simulink model "rx2"  (R2022b)
settings: Solver=FixedStepDiscrete  StartTime=0.0  StopTime=3.3E6  FixedStep=1  RelTol=1e-3  EnableMultiTasking=on
model workspace (MAT data in the model file):
  mwTaskManagerKernelLatency = 0
undefined symbols (not defined in the file or in its folder): Add, jsin, magnitude, rom_pilot_conj_tt, Shift
libraries: hdlsllib x3231, whdlutilities x525, simulink x260, whdlmod x112, whdledac x26, dsphdlmathfun2 x24, commchan3 x1
(part 39 of 59)

== system rx2/demode1/chan_est1/Subsystem/HDL_DUT1/H_est ==
  H_result_in : Inport
      settings: SignalType=complex
  H_ctrl_in : Inport  Port=2  OutDataTypeStr=Bus: samplecontrol
  Complex to Real-Imag : ComplexToRealImag
  Constant1 : Constant  OutDataTypeStr=fixdt(1,33,28)
  Constant2 : Constant  Value=2  OutDataTypeStr=uint8
  Counter1 : hdlsllib/Sources/HDL Counter  CountType=Count limited  CountInit=0  CountStep=1  CountMax=1  CountFromType=Initial value  CountFrom=0  CountResetPort=off  CountLoadPort=off  CountEnbPort=on  CountDirPort=off  CountHitOutputPort=off  CountDataType=Unsigned  CountWordLen=8  CountFracLen=0  CountSampTime=1
  Counter2 : hdlsllib/Sources/HDL Counter  CountType=Count limited  CountInit=0  CountStep=1  CountMax=511  CountFromType=Initial value  CountFrom=0  CountResetPort=off  CountLoadPort=off  CountEnbPort=on  CountDirPort=off  CountHitOutputPort=off  CountDataType=Unsigned  CountWordLen=16  CountFracLen=0  CountSampTime=1
  Counter3 : hdlsllib/Sources/HDL Counter  CountType=Count limited  CountInit=0  CountStep=1  CountMax=511  CountFromType=Initial value  CountFrom=0  CountResetPort=on  CountLoadPort=off  CountEnbPort=on  CountDirPort=off  CountHitOutputPort=off  CountDataType=Unsigned  CountWordLen=16  CountFracLen=0  CountSampTime=1
  Counter4 : hdlsllib/Sources/HDL Counter  CountType=Count limited  CountInit=0  CountStep=1  CountMax=5  CountFromType=Initial value  CountFrom=0  CountResetPort=on  CountLoadPort=off  CountEnbPort=on  CountDirPort=off  CountHitOutputPort=on  CountDataType=Unsigned  CountWordLen=16  CountFracLen=0  CountSampTime=1
  Delay1 : Delay  DelayLength=1  InitialCondition=0
  Delay2 : Delay  DelayLength=12  InitialCondition=0
  Delay3 : Delay  DelayLength=1  InitialCondition=0
  Delay4 : Delay  DelayLength=1  InitialCondition=0
  Delay5 : Delay  DelayLength=12  InitialCondition=0
  Delay6 : Delay  DelayLength=12  InitialCondition=0
  Gain3 : Gain  Gain=1/6  OutDataTypeStr=fixdt(1,32,27)
  Ground{1..6} (6 alike) : Ground
  Logical Operator : Logic  Operator=XOR  AllPortsSameDT=off  OutDataTypeStr=boolean
  Logical Operator2 : Logic  Operator=OR  AllPortsSameDT=off  OutDataTypeStr=boolean
  Mod : Math  Operator=mod  SignedPower=on
  MultiplyAccumulate : hdlsllib/HDL Operations/Multiply-Accumulate  opMode=Streaming - using Number of Samples  initValueSetting=Dialog  initValue=0  initValueSetting2=Dialog  initValue2=0  initValueSetting3=Dialog  initValue3=0  num_samples=6  RndMeth2=Floor  RndMeth3=Floor  datatype2=Inherit: Inherit via back propagation  datatype3=Inherit: Inherit via back propagation  validOut=on  endInandOut=on  startOut=on  countOut=on  dim=-1  DoSatur=off  parallel=off
  MultiplyAccumulate1 : hdlsllib/HDL Operations/Multiply-Accumulate  opMode=Streaming - using Number of Samples  initValueSetting=Dialog  initValue=0  initValueSetting2=Dialog  initValue2=0  initValueSetting3=Dialog  initValue3=0  num_samples=6  RndMeth2=Floor  RndMeth3=Floor  datatype2=Inherit: Inherit via back propagation  datatype3=Inherit: Inherit via back propagation  validOut=on  endInandOut=on  startOut=on  countOut=on  dim=-1  DoSatur=off  parallel=off
  Real-Imag to Complex : RealImagToComplex
  Sample Control Bus Creator : whdlutilities/Sample Control Bus Creator
  Sample Control Bus Selector : whdlutilities/Sample Control Bus Selector  OutputSignals=start,end,valid
  Switch1 : Switch  Threshold=396  SaturateOnIntegerOverflow=off  InputSameDT=off
  Switch2 : Switch  Threshold=1  SaturateOnIntegerOverflow=off  InputSameDT=off
  Switch3 : Switch  Threshold=5  SaturateOnIntegerOverflow=off  InputSameDT=off
  Switch4 : Switch  Threshold=396  SaturateOnIntegerOverflow=off  InputSameDT=off
  Switch5 : Switch  Threshold=396  SaturateOnIntegerOverflow=off  InputSameDT=off
  Switch6 : Switch  Threshold=5  SaturateOnIntegerOverflow=off  InputSameDT=off
  hRAM1 : Subsystem
  H_out : Outport  VectorParamsAs1DForOutWhenUnconnected=off
  H_valid_out : Outport  Port=2  VectorParamsAs1DForOutWhenUnconnected=off
  wires:
  Switch4/1 -> Switch3/1  "H_sum"
  Sample Control Bus Selector/2 -> Logical Operator2/1, Delay4/1
  Sample Control Bus Selector/1 -> Delay3/1, Logical Operator2/2, Counter3/1
  Logical Operator/1 -> Switch2/2, Switch1/3, Counter3/2, Counter2/1  "valid_1024"
  Switch2/1 -> MultiplyAccumulate/1
  Counter1/1 -> Mod/1
  Ground1/1 -> Switch2/3
  Counter3/1 -> Switch5/2, Switch4/2
  Ground4/1 -> Switch1/1
  Ground2/1 -> Switch3/3
  MultiplyAccumulate/1 -> Switch4/3
  H_ctrl_in/1 -> Sample Control Bus Selector/1
  Delay1/1 -> Delay5/1, hRAM1/2(H_valid_out)
  Ground3/1 -> Switch4/1
  Logical Operator2/1 -> Counter4/1
  Switch1/1 -> MultiplyAccumulate1/3, MultiplyAccumulate/3, Counter4/2  "valid_792"
  Constant2/1 -> Mod/2
  Counter4/1 -> Switch6/2, Switch3/2
  Counter2/1 -> Switch1/2
  Delay3/1 -> Delay2/1
  Mod/1 -> Logical Operator/2
  Constant1/1 -> MultiplyAccumulate1/2, MultiplyAccumulate/2
  Delay4/1 -> hRAM1/3(H_end_out), Delay6/1
  hRAM1/1(Out1) -> H_out/1
  Sample Control Bus Selector/3 -> Counter1/1, Logical Operator/1, Delay1/1
  Sample Control Bus Creator/1 -> H_valid_out/1
  H_result_in/1 -> Complex to Real-Imag/1
  MultiplyAccumulate1/1 -> Switch5/3
  Ground5/1 -> Switch5/1
  Switch5/1 -> Switch6/1  "H_sum"
  Ground6/1 -> Switch6/3
  Complex to Real-Imag/1 -> MultiplyAccumulate1/1
  Complex to Real-Imag/2 -> Switch2/1
  Gain3/1 -> hRAM1/1(H_out)  "average"
  Switch6/1 -> Real-Imag to Complex/1
  Switch3/1 -> Real-Imag to Complex/2
  Real-Imag to Complex/1 -> Gain3/1
  Delay2/1 -> Sample Control Bus Creator/1
  Delay5/1 -> Sample Control Bus Creator/3
  Delay6/1 -> Sample Control Bus Creator/2

== system rx2/demode1/chan_est1/Subsystem/HDL_DUT1/LS_Est ==
  LS_data_in : Inport
  LS_polit_in : Inport  Port=2  OutDataTypeStr=fixdt(1,16,14)
  LS_valid_in : Inport  Port=3
  Complex to Magnitude-Angle : dsphdlmathfun2/Complex to Magnitude-Angle  NumIterationsSource=Property  NumIterations=10  OutputFormat=Magnitude and angle  AngleFormat=Normalized  ScaleOutput=on  ScalingMethod=Multiplier  SimulateUsing=Code generation
  Complex to Magnitude-Angle1 : dsphdlmathfun2/Complex to Magnitude-Angle  NumIterationsSource=Property  NumIterations=10  OutputFormat=Magnitude and angle  AngleFormat=Normalized  ScaleOutput=on  ScalingMethod=Shift-Add  SimulateUsing=Code generation
  Dot Product : DotProduct  OutDataTypeStr=fixdt(1,16,12)
  Ground : Ground
  Ground1 : Ground
  HDL Counter : hdlsllib/Sources/HDL Counter  CountType=Count limited  CountInit=0  CountStep=1  CountMax=1  CountFromType=Initial value  CountFrom=0  CountResetPort=off  CountLoadPort=off  CountEnbPort=on  CountDirPort=off  CountHitOutputPort=off  CountDataType=Unsigned  CountWordLen=2  CountFracLen=0  CountSampTime=1
  Switch1 : Switch  Threshold=1  OutDataTypeStr=fixdt(1,16,14)  SaturateOnIntegerOverflow=off  InputSameDT=off
  Switch2 : Switch  Threshold=1  OutDataTypeStr=fixdt(1,16,14)  SaturateOnIntegerOverflow=off  InputSameDT=off
  ctrl_gen : Subsystem
  ctrl_gen1 : Subsystem
  LS_result_out : Outport  VectorParamsAs1DForOutWhenUnconnected=off
  LS_ctrl_out : Outport  Port=2  VectorParamsAs1DForOutWhenUnconnected=off
  wdata_out : Outport  Port=3  VectorParamsAs1DForOutWhenUnconnected=off
  wvalid_out : Outport  Port=4  VectorParamsAs1DForOutWhenUnconnected=off
  wires:
  LS_data_in/1 -> Switch1/1, Switch2/1
  Switch1/1 -> Dot Product/1  "data"
  Dot Product/1 -> Complex to Magnitude-Angle/1
  Ground/1 -> Switch1/3
  LS_valid_in/1 -> Complex to Magnitude-Angle/2, Complex to Magnitude-Angle1/2, HDL Counter/1, Switch1/2
  LS_polit_in/1 -> Dot Product/2
  Complex to Magnitude-Angle/1 -> ctrl_gen/1(data_in)  "result"
  Complex to Magnitude-Angle/3 -> ctrl_gen/2(valid_in)  "valid2"
  ctrl_gen/1(data_out) -> LS_result_out/1
  ctrl_gen/2(ctrl_out) -> LS_ctrl_out/1
  HDL Counter/1 -> Switch2/2
  Ground1/1 -> Switch2/3
  Switch2/1 -> Complex to Magnitude-Angle1/1  "data"
  Complex to Magnitude-Angle1/1 -> wdata_out/1
  Complex to Magnitude-Angle1/3 -> ctrl_gen1/1(valid_in)
  ctrl_gen1/1(wvalid_out) -> wvalid_out/1

== system rx2/demode1/chan_est1/Subsystem/HDL_DUT1/Pliot ==
  enb : Inport
  Counter1 : hdlsllib/Sources/HDL Counter  CountType=Count limited  CountInit=0  CountStep=1  CountMax=7  CountFromType=Initial value  CountFrom=0  CountResetPort=off  CountLoadPort=off  CountEnbPort=on  CountDirPort=off  CountHitOutputPort=off  CountDataType=Unsigned  CountWordLen=8  CountFracLen=0  CountSampTime=1
  Data Type Conversion3 : DataTypeConversion  OutDataTypeStr=uint8  SaturateOnIntegerOverflow=off  RndMeth=Floor
  rom : Subsystem
  pilot : Outport
  wires:
  enb/1 -> Counter1/1
  Counter1/1 -> Data Type Conversion3/1
  Data Type Conversion3/1 -> rom/1(address)
  rom/1(data_out) -> pilot/1  "pilot"

== system rx2/demode1/chan_est1/Subsystem/HDL_DUT1/TA_EST ==
  data_in : Inport
  ctrl_in : Inport  Port=2  OutDataTypeStr=Bus: samplecontrol
  Bus Selector : BusSelector  OutputSignals=start,end,valid
  Complex to Magnitude-Angle : dsphdlmathfun2/Complex to Magnitude-Angle  NumIterationsSource=Property  NumIterations=10  OutputFormat=Magnitude and angle  AngleFormat=Radians  ScaleOutput=on  ScalingMethod=Shift-Add  SimulateUsing=Code generation
  Constant : Constant  OutDataTypeStr=fixdt(1,34,24)
  Counter1 : hdlsllib/Sources/HDL Counter  CountType=Count limited  CountInit=0  CountStep=1  CountMax=1  CountFromType=Initial value  CountFrom=0  CountResetPort=off  CountLoadPort=off  CountEnbPort=on  CountDirPort=off  CountHitOutputPort=off  CountDataType=Unsigned  CountWordLen=8  CountFracLen=0  CountSampTime=1
  Counter2 : hdlsllib/Sources/HDL Counter  CountType=Count limited  CountInit=0  CountStep=1  CountMax=511  CountFromType=Initial value  CountFrom=0  CountResetPort=off  CountLoadPort=off  CountEnbPort=on  CountDirPort=off  CountHitOutputPort=off  CountDataType=Unsigned  CountWordLen=16  CountFracLen=0  CountSampTime=1
  Counter3 : hdlsllib/Sources/HDL Counter  CountType=Count limited  CountInit=0  CountStep=1  CountMax=5  CountFromType=Initial value  CountFrom=0  CountResetPort=off  CountLoadPort=off  CountEnbPort=on  CountDirPort=off  CountHitOutputPort=on  CountDataType=Unsigned  CountWordLen=8  CountFracLen=0  CountSampTime=1
  Counter4 : hdlsllib/Sources/HDL Counter  CountType=Count limited  CountInit=0  CountStep=1  CountMax=395  CountFromType=Initial value  CountFrom=0  CountResetPort=off  CountLoadPort=off  CountEnbPort=on  CountDirPort=off  CountHitOutputPort=off  CountDataType=Unsigned  CountWordLen=16  CountFracLen=0  CountSampTime=1
  Data Type Conversion : DataTypeConversion  OutDataTypeStr=boolean  SaturateOnIntegerOverflow=off  RndMeth=Floor
  Data Type Conversion1 : DataTypeConversion  OutDataTypeStr=fixdt(1,26,14)  SaturateOnIntegerOverflow=off  RndMeth=Floor
  Data Type Conversion2 : DataTypeConversion  OutDataTypeStr=fixdt(1,26,14)  SaturateOnIntegerOverflow=off  RndMeth=Floor
  Data Type Conversion3 : DataTypeConversion  OutDataTypeStr=fixdt(1,16,14)  SaturateOnIntegerOverflow=off  RndMeth=Floor
  Delay1 : Delay  InitialCondition=0
  Delay2 : Delay  InitialCondition=0
  Delay3 : Delay  DelayLength=1  InitialCondition=0
  Delay4 : Delay  DelayLength=3  InitialCondition=0
  Delay5 : Delay  DelayLength=18  InitialCondition=0
  Delay6 : Delay  DelayLength=15  InitialCondition=0
  Delay7 : Delay  DelayLength=1  InitialCondition=0
  Dot Product : DotProduct  OutDataTypeStr=Inherit: Inherit via internal rule
  Dot Product1 : DotProduct  OutDataTypeStr=fixdt(1,26,14)
  Ground : Ground
  Ground4 : Ground
  Logical Operator : Logic  Operator=XOR  AllPortsSameDT=off  OutDataTypeStr=boolean
  Logical Operator1 : Logic  AllPortsSameDT=off  OutDataTypeStr=boolean
  Logical Operator2 : Logic  Operator=XOR  AllPortsSameDT=off  OutDataTypeStr=boolean
  Multiply-Accumulate : hdlsllib/HDL Operations/Multiply-Accumulate  opMode=Streaming - using Number of Samples  initValueSetting=Dialog  initValue=0  initValueSetting2=Dialog  initValue2=0  initValueSetting3=Dialog  initValue3=0  num_samples=330  RndMeth2=Floor  RndMeth3=Floor  datatype2=Inherit: Inherit via back propagation  datatype3=fixdt(1,68,48)  validOut=on  endInandOut=on  startOut=on  countOut=on  dim=-1  DoSatur=off  parallel=off
  Product : Product
  Switch : Switch  Criteria=u2 ~= 0  OutDataTypeStr=fixdt(1,26,14)  SaturateOnIntegerOverflow=off  InputSameDT=off
  Switch1 : Switch  Threshold=396  SaturateOnIntegerOverflow=off  InputSameDT=off
  cos + jsin : Trigonometry  Operator=cos + jsin  ApproximationMethod=CORDIC  NumberOfIterations=10
  ctrl_gen : Subsystem
  hta_est_data : Outport  VectorParamsAs1DForOutWhenUnconnected=off
  hta_est_ctrl : Outport  Port=2  VectorParamsAs1DForOutWhenUnconnected=off
  wires:
  ctrl_in/1 -> Bus Selector/1
  data_in/1 -> Delay5/1, Dot Product/1, Delay1/1
  Dot Product/1 -> Multiply-Accumulate/1
  Delay1/1 -> Dot Product/2
  Constant/1 -> Multiply-Accumulate/2
  Multiply-Accumulate/1 -> Complex to Magnitude-Angle/1
  Ground4/1 -> Switch1/1
  Counter2/1 -> Switch1/2
  Logical Operator/1 -> Switch1/3, Counter2/1  "valid_1024"
  Counter1/1 -> Data Type Conversion/1
  Delay2/1 -> Logical Operator/1, Counter1/1
  Switch1/1 -> Delay6/1, Logical Operator2/1, Counter3/1  "valid_792"
  Data Type Conversion/1 -> Logical Operator/2
  Counter3/2 -> Logical Operator1/2, Delay3/1
  Delay3/1 -> Logical Operator1/1
  Logical Operator1/1 -> Logical Operator2/2
  Logical Operator2/1 -> Multiply-Accumulate/3
  Delay4/1 -> Complex to Magnitude-Angle/2
  Complex to Magnitude-Angle/3 -> Delay7/1
  Delay6/1 -> Counter4/1
  Complex to Magnitude-Angle/2 -> Data Type Conversion2/1
  Counter4/1 -> Data Type Conversion1/1
  Data Type Conversion1/1 -> Dot Product1/2
  Dot Product1/1 -> Data Type Conversion3/1
  Data Type Conversion2/1 -> Dot Product1/1
  Switch/1 -> Product/2
  Ground/1 -> Switch/3
  Delay7/1 -> ctrl_gen/2(valid_in), Switch/2
  Delay5/1 -> Product/1
  Bus Selector/3 -> [valid], Delay4/1, Delay2/1  "<valid>"
  ctrl_gen/2(ctrl_out) -> hta_est_ctrl/1  "OFDM_ctrl_bf1_process1"
  ctrl_gen/1(data_out) -> hta_est_data/1  "OFDM_bf1_process1"
  Product/1 -> ctrl_gen/1(data_in)
  cos + jsin/1 -> Switch/1
  Data Type Conversion3/1 -> cos + jsin/1

== system rx2/demode1/chan_est1/Subsystem/HDL_DUT1/delta_estimator ==
  data_in : Inport
  valid_in : Inport  Port=2  OutDataTypeStr=boolean
  Add1 : Sum  Inputs=+-  AccumDataTypeStr=fixdt(1,64,56)  OutDataTypeStr=fixdt(1,32,28)
  Delay2 : Delay  DelayLength=1  InitialCondition=0
  calculate_norm2 : Subsystem
  calculate_norm3 : Subsystem
  iteration_estimation : Subsystem
  iteration_estimation1 : Subsystem
  data_out : Outport  OutDataTypeStr=fixdt(1,16,14)  VectorParamsAs1DForOutWhenUnconnected=off
  valid_out : Outport  Port=2  OutDataTypeStr=boolean  VectorParamsAs1DForOutWhenUnconnected=off
  wires:
  valid_in/1 -> iteration_estimation/2(valid_in)
  iteration_estimation/1(data_out) -> calculate_norm3/1(data_in)
  calculate_norm2/1(data_out) -> Add1/1
  calculate_norm3/1(data_out) -> Add1/2
  Add1/1 -> iteration_estimation1/1(data_in)
  data_in/1 -> Delay2/1, iteration_estimation/1(data_in)
  iteration_estimation1/1(data_out) -> data_out/1
  iteration_estimation1/2(valid_out) -> valid_out/1
  Delay2/1 -> calculate_norm2/1(data_in)
  iteration_estimation/2(valid_out) -> iteration_estimation1/2(valid_in)

== system rx2/demode1/chan_est1/Subsystem/HDL_DUT2/H_est ==
  H_result_in : Inport
      settings: SignalType=complex
  H_ctrl_in : Inport  Port=2  OutDataTypeStr=Bus: samplecontrol
  Complex to Real-Imag : ComplexToRealImag
  Constant1 : Constant  OutDataTypeStr=fixdt(1,33,28)
  Constant2 : Constant  Value=2  OutDataTypeStr=uint8
  Counter1 : hdlsllib/Sources/HDL Counter  CountType=Count limited  CountInit=0  CountStep=1  CountMax=1  CountFromType=Initial value  CountFrom=0  CountResetPort=off  CountLoadPort=off  CountEnbPort=on  CountDirPort=off  CountHitOutputPort=off  CountDataType=Unsigned  CountWordLen=8  CountFracLen=0  CountSampTime=1
  Counter2 : hdlsllib/Sources/HDL Counter  CountType=Count limited  CountInit=0  CountStep=1  CountMax=511  CountFromType=Initial value  CountFrom=0  CountResetPort=off  CountLoadPort=off  CountEnbPort=on  CountDirPort=off  CountHitOutputPort=off  CountDataType=Unsigned  CountWordLen=16  CountFracLen=0  CountSampTime=1
  Counter3 : hdlsllib/Sources/HDL Counter  CountType=Count limited  CountInit=0  CountStep=1  CountMax=511  CountFromType=Initial value  CountFrom=0  CountResetPort=on  CountLoadPort=off  CountEnbPort=on  CountDirPort=off  CountHitOutputPort=off  CountDataType=Unsigned  CountWordLen=16  CountFracLen=0  CountSampTime=1
  Counter4 : hdlsllib/Sources/HDL Counter  CountType=Count limited  CountInit=0  CountStep=1  CountMax=5  CountFromType=Initial value  CountFrom=0  CountResetPort=on  CountLoadPort=off  CountEnbPort=on  CountDirPort=off  CountHitOutputPort=on  CountDataType=Unsigned  CountWordLen=16  CountFracLen=0  CountSampTime=1
  Delay1 : Delay  DelayLength=1  InitialCondition=0
  Delay2 : Delay  DelayLength=12  InitialCondition=0
  Delay3 : Delay  DelayLength=1  InitialCondition=0
  Delay4 : Delay  DelayLength=1  InitialCondition=0
  Delay5 : Delay  DelayLength=12  InitialCondition=0
  Delay6 : Delay  DelayLength=12  InitialCondition=0
  Gain3 : Gain  Gain=1/6  OutDataTypeStr=fixdt(1,32,27)
  Ground{1..6} (6 alike) : Ground
  Logical Operator : Logic  Operator=XOR  AllPortsSameDT=off  OutDataTypeStr=boolean
  Logical Operator2 : Logic  Operator=OR  AllPortsSameDT=off  OutDataTypeStr=boolean
  Mod : Math  Operator=mod  SignedPower=on
  MultiplyAccumulate : hdlsllib/HDL Operations/Multiply-Accumulate  opMode=Streaming - using Number of Samples  initValueSetting=Dialog  initValue=0  initValueSetting2=Dialog  initValue2=0  initValueSetting3=Dialog  initValue3=0  num_samples=6  RndMeth2=Floor  RndMeth3=Floor  datatype2=Inherit: Inherit via back propagation  datatype3=Inherit: Inherit via back propagation  validOut=on  endInandOut=on  startOut=on  countOut=on  dim=-1  DoSatur=off  parallel=off
  MultiplyAccumulate1 : hdlsllib/HDL Operations/Multiply-Accumulate  opMode=Streaming - using Number of Samples  initValueSetting=Dialog  initValue=0  initValueSetting2=Dialog  initValue2=0  initValueSetting3=Dialog  initValue3=0  num_samples=6  RndMeth2=Floor  RndMeth3=Floor  datatype2=Inherit: Inherit via back propagation  datatype3=Inherit: Inherit via back propagation  validOut=on  endInandOut=on  startOut=on  countOut=on  dim=-1  DoSatur=off  parallel=off
  Real-Imag to Complex : RealImagToComplex
  Sample Control Bus Creator : whdlutilities/Sample Control Bus Creator
  Sample Control Bus Selector : whdlutilities/Sample Control Bus Selector  OutputSignals=start,end,valid
  Switch1 : Switch  Threshold=396  SaturateOnIntegerOverflow=off  InputSameDT=off
  Switch2 : Switch  Threshold=1  SaturateOnIntegerOverflow=off  InputSameDT=off
  Switch3 : Switch  Threshold=5  SaturateOnIntegerOverflow=off  InputSameDT=off
  Switch4 : Switch  Threshold=396  SaturateOnIntegerOverflow=off  InputSameDT=off
  Switch5 : Switch  Threshold=396  SaturateOnIntegerOverflow=off  InputSameDT=off
  Switch6 : Switch  Threshold=5  SaturateOnIntegerOverflow=off  InputSameDT=off
  hRAM1 : Subsystem
  H_out : Outport  VectorParamsAs1DForOutWhenUnconnected=off
  H_valid_out : Outport  Port=2  VectorParamsAs1DForOutWhenUnconnected=off
  wires:
  Switch4/1 -> Switch3/1  "H_sum"
  Sample Control Bus Selector/2 -> Logical Operator2/1, Delay4/1
  Sample Control Bus Selector/1 -> Delay3/1, Logical Operator2/2, Counter3/1
  Logical Operator/1 -> Switch2/2, Switch1/3, Counter3/2, Counter2/1  "valid_1024"
  Switch2/1 -> MultiplyAccumulate/1
  Counter1/1 -> Mod/1
  Ground1/1 -> Switch2/3
  Counter3/1 -> Switch5/2, Switch4/2
  Ground4/1 -> Switch1/1
  Ground2/1 -> Switch3/3
  MultiplyAccumulate/1 -> Switch4/3
  H_ctrl_in/1 -> Sample Control Bus Selector/1
  Delay1/1 -> Delay5/1, hRAM1/2(H_valid_out)
  Ground3/1 -> Switch4/1
  Logical Operator2/1 -> Counter4/1
  Switch1/1 -> MultiplyAccumulate1/3, MultiplyAccumulate/3, Counter4/2  "valid_792"
  Constant2/1 -> Mod/2
  Counter4/1 -> Switch6/2, Switch3/2
  Counter2/1 -> Switch1/2
  Delay3/1 -> Delay2/1
  Mod/1 -> Logical Operator/2
  Constant1/1 -> MultiplyAccumulate1/2, MultiplyAccumulate/2
  Delay4/1 -> hRAM1/3(H_end_out), Delay6/1
  hRAM1/1(Out1) -> H_out/1
  Sample Control Bus Selector/3 -> Counter1/1, Logical Operator/1, Delay1/1
  Sample Control Bus Creator/1 -> H_valid_out/1
  H_result_in/1 -> Complex to Real-Imag/1
  MultiplyAccumulate1/1 -> Switch5/3
  Ground5/1 -> Switch5/1
  Switch5/1 -> Switch6/1  "H_sum"
  Ground6/1 -> Switch6/3
  Complex to Real-Imag/1 -> MultiplyAccumulate1/1
  Complex to Real-Imag/2 -> Switch2/1
  Gain3/1 -> hRAM1/1(H_out)  "average"
  Switch6/1 -> Real-Imag to Complex/1
  Switch3/1 -> Real-Imag to Complex/2
  Real-Imag to Complex/1 -> Gain3/1
  Delay2/1 -> Sample Control Bus Creator/1
  Delay5/1 -> Sample Control Bus Creator/3
  Delay6/1 -> Sample Control Bus Creator/2

== system rx2/demode1/chan_est1/Subsystem/HDL_DUT2/LS_Est ==
  LS_data_in : Inport
  LS_polit_in : Inport  Port=2  OutDataTypeStr=fixdt(1,16,14)
  LS_valid_in : Inport  Port=3
  Complex to Magnitude-Angle : dsphdlmathfun2/Complex to Magnitude-Angle  NumIterationsSource=Property  NumIterations=10  OutputFormat=Magnitude and angle  AngleFormat=Normalized  ScaleOutput=on  ScalingMethod=Multiplier  SimulateUsing=Code generation
  Complex to Magnitude-Angle1 : dsphdlmathfun2/Complex to Magnitude-Angle  NumIterationsSource=Property  NumIterations=10  OutputFormat=Magnitude and angle  AngleFormat=Normalized  ScaleOutput=on  ScalingMethod=Shift-Add  SimulateUsing=Code generation
  Dot Product : DotProduct  OutDataTypeStr=fixdt(1,16,12)
  Ground : Ground
  Ground1 : Ground
  HDL Counter : hdlsllib/Sources/HDL Counter  CountType=Count limited  CountInit=0  CountStep=1  CountMax=1  CountFromType=Initial value  CountFrom=0  CountResetPort=off  CountLoadPort=off  CountEnbPort=on  CountDirPort=off  CountHitOutputPort=off  CountDataType=Unsigned  CountWordLen=2  CountFracLen=0  CountSampTime=1
  Switch1 : Switch  Threshold=1  OutDataTypeStr=fixdt(1,16,14)  SaturateOnIntegerOverflow=off  InputSameDT=off
  Switch2 : Switch  Threshold=1  OutDataTypeStr=fixdt(1,16,14)  SaturateOnIntegerOverflow=off  InputSameDT=off
  ctrl_gen : Subsystem
  ctrl_gen1 : Subsystem
  LS_result_out : Outport  VectorParamsAs1DForOutWhenUnconnected=off
  LS_ctrl_out : Outport  Port=2  VectorParamsAs1DForOutWhenUnconnected=off
  wdata_out : Outport  Port=3  VectorParamsAs1DForOutWhenUnconnected=off
  wvalid_out : Outport  Port=4  VectorParamsAs1DForOutWhenUnconnected=off
  wires:
  LS_data_in/1 -> Switch1/1, Switch2/1
  Switch1/1 -> Dot Product/1  "data"
  Dot Product/1 -> Complex to Magnitude-Angle/1
  Ground/1 -> Switch1/3
  LS_valid_in/1 -> Complex to Magnitude-Angle/2, Complex to Magnitude-Angle1/2, Switch1/2
  LS_polit_in/1 -> Dot Product/2
  Complex to Magnitude-Angle/1 -> ctrl_gen/1(data_in)  "result"
  Complex to Magnitude-Angle/3 -> ctrl_gen/2(valid_in)  "valid2"
  ctrl_gen/1(data_out) -> LS_result_out/1
  ctrl_gen/2(ctrl_out) -> LS_ctrl_out/1
  HDL Counter/1 -> Switch2/2
  Ground1/1 -> Switch2/3
  Switch2/1 -> Complex to Magnitude-Angle1/1  "data"
  Complex to Magnitude-Angle1/1 -> wdata_out/1
  Complex to Magnitude-Angle1/3 -> ctrl_gen1/1(valid_in)
  ctrl_gen1/1(wvalid_out) -> wvalid_out/1

== system rx2/demode1/chan_est1/Subsystem/HDL_DUT2/Pliot ==
  enb : Inport
  Counter1 : hdlsllib/Sources/HDL Counter  CountType=Count limited  CountInit=0  CountStep=1  CountMax=7  CountFromType=Initial value  CountFrom=0  CountResetPort=off  CountLoadPort=off  CountEnbPort=on  CountDirPort=off  CountHitOutputPort=off  CountDataType=Unsigned  CountWordLen=8  CountFracLen=0  CountSampTime=1
  Data Type Conversion3 : DataTypeConversion  OutDataTypeStr=uint8  SaturateOnIntegerOverflow=off  RndMeth=Floor
  rom : Subsystem
  pilot : Outport
  wires:
  enb/1 -> ?
  Counter1/1 -> Data Type Conversion3/1
  Data Type Conversion3/1 -> rom/1(address)
  rom/1(data_out) -> pilot/1  "pilot"

== system rx2/demode1/chan_est1/Subsystem/HDL_DUT2/TA_EST ==
  data_in : Inport
  ctrl_in : Inport  Port=2  OutDataTypeStr=Bus: samplecontrol
  Bus Selector : BusSelector  OutputSignals=start,end,valid
  Complex to Magnitude-Angle : dsphdlmathfun2/Complex to Magnitude-Angle  NumIterationsSource=Property  NumIterations=10  OutputFormat=Magnitude and angle  AngleFormat=Radians  ScaleOutput=on  ScalingMethod=Shift-Add  SimulateUsing=Code generation
  Constant : Constant  OutDataTypeStr=fixdt(1,34,24)
  Counter1 : hdlsllib/Sources/HDL Counter  CountType=Count limited  CountInit=0  CountStep=1  CountMax=1  CountFromType=Initial value  CountFrom=0  CountResetPort=off  CountLoadPort=off  CountEnbPort=on  CountDirPort=off  CountHitOutputPort=off  CountDataType=Unsigned  CountWordLen=8  CountFracLen=0  CountSampTime=1
  Counter2 : hdlsllib/Sources/HDL Counter  CountType=Count limited  CountInit=0  CountStep=1  CountMax=511  CountFromType=Initial value  CountFrom=0  CountResetPort=off  CountLoadPort=off  CountEnbPort=on  CountDirPort=off  CountHitOutputPort=off  CountDataType=Unsigned  CountWordLen=16  CountFracLen=0  CountSampTime=1
  Counter3 : hdlsllib/Sources/HDL Counter  CountType=Count limited  CountInit=0  CountStep=1  CountMax=5  CountFromType=Initial value  CountFrom=0  CountResetPort=off  CountLoadPort=off  CountEnbPort=on  CountDirPort=off  CountHitOutputPort=on  CountDataType=Unsigned  CountWordLen=8  CountFracLen=0  CountSampTime=1
  Counter4 : hdlsllib/Sources/HDL Counter  CountType=Count limited  CountInit=0  CountStep=1  CountMax=395  CountFromType=Initial value  CountFrom=0  CountResetPort=off  CountLoadPort=off  CountEnbPort=on  CountDirPort=off  CountHitOutputPort=off  CountDataType=Unsigned  CountWordLen=16  CountFracLen=0  CountSampTime=1
  Data Type Conversion : DataTypeConversion  OutDataTypeStr=boolean  SaturateOnIntegerOverflow=off  RndMeth=Floor
  Data Type Conversion1 : DataTypeConversion  OutDataTypeStr=fixdt(1,26,14)  SaturateOnIntegerOverflow=off  RndMeth=Floor
  Data Type Conversion2 : DataTypeConversion  OutDataTypeStr=fixdt(1,26,14)  SaturateOnIntegerOverflow=off  RndMeth=Floor
  Data Type Conversion3 : DataTypeConversion  OutDataTypeStr=fixdt(1,16,14)  SaturateOnIntegerOverflow=off  RndMeth=Floor
  Delay1 : Delay  InitialCondition=0
  Delay2 : Delay  InitialCondition=0
  Delay3 : Delay  DelayLength=1  InitialCondition=0
  Delay4 : Delay  DelayLength=3  InitialCondition=0
  Delay5 : Delay  DelayLength=18  InitialCondition=0
  Delay6 : Delay  DelayLength=15  InitialCondition=0
  Delay7 : Delay  DelayLength=1  InitialCondition=0
  Dot Product : DotProduct  OutDataTypeStr=Inherit: Inherit via internal rule
  Dot Product1 : DotProduct  OutDataTypeStr=fixdt(1,26,14)
  Ground : Ground
  Ground4 : Ground
  Logical Operator : Logic  Operator=XOR  AllPortsSameDT=off  OutDataTypeStr=boolean
  Logical Operator1 : Logic  AllPortsSameDT=off  OutDataTypeStr=boolean
  Logical Operator2 : Logic  Operator=XOR  AllPortsSameDT=off  OutDataTypeStr=boolean
  Multiply-Accumulate : hdlsllib/HDL Operations/Multiply-Accumulate  opMode=Streaming - using Number of Samples  initValueSetting=Dialog  initValue=0  initValueSetting2=Dialog  initValue2=0  initValueSetting3=Dialog  initValue3=0  num_samples=330  RndMeth2=Floor  RndMeth3=Floor  datatype2=Inherit: Inherit via back propagation  datatype3=fixdt(1,68,48)  validOut=on  endInandOut=on  startOut=on  countOut=on  dim=-1  DoSatur=off  parallel=off
  Product : Product
  Switch : Switch  Criteria=u2 ~= 0  OutDataTypeStr=fixdt(1,26,14)  SaturateOnIntegerOverflow=off  InputSameDT=off
  Switch1 : Switch  Threshold=396  SaturateOnIntegerOverflow=off  InputSameDT=off
  cos + jsin : Trigonometry  Operator=cos + jsin  ApproximationMethod=CORDIC  NumberOfIterations=10
  ctrl_gen : Subsystem
  hta_est_data : Outport  VectorParamsAs1DForOutWhenUnconnected=off
  hta_est_ctrl : Outport  Port=2  VectorParamsAs1DForOutWhenUnconnected=off
  wires:
  ctrl_in/1 -> Bus Selector/1
  data_in/1 -> Delay5/1, Dot Product/1, Delay1/1
  Dot Product/1 -> Multiply-Accumulate/1
  Delay1/1 -> Dot Product/2
  Constant/1 -> Multiply-Accumulate/2
  Multiply-Accumulate/1 -> Complex to Magnitude-Angle/1
  Ground4/1 -> Switch1/1
  Counter2/1 -> Switch1/2
  Logical Operator/1 -> Switch1/3  "valid_1024"
  Counter1/1 -> Data Type Conversion/1
  Delay2/1 -> Logical Operator/1
  Switch1/1 -> Delay6/1, Logical Operator2/1  "valid_792"
  Data Type Conversion/1 -> Logical Operator/2
  ? -> Logical Operator1/2, Delay3/1
  Delay3/1 -> Logical Operator1/1
  Logical Operator1/1 -> Logical Operator2/2
  Logical Operator2/1 -> ?
  Delay4/1 -> Complex to Magnitude-Angle/2
  Complex to Magnitude-Angle/3 -> Delay7/1
  Delay6/1 -> ?
  Complex to Magnitude-Angle/2 -> Data Type Conversion2/1
  Counter4/1 -> Data Type Conversion1/1
  Data Type Conversion1/1 -> Dot Product1/2
  Dot Product1/1 -> Data Type Conversion3/1
  Data Type Conversion2/1 -> Dot Product1/1
  Switch/1 -> Product/2
  Ground/1 -> Switch/3
  Delay7/1 -> ctrl_gen/2(valid_in), Switch/2
  Delay5/1 -> Product/1
  Bus Selector/3 -> [valid], Delay4/1, Delay2/1  "<valid>"
  ctrl_gen/2(ctrl_out) -> hta_est_ctrl/1  "OFDM_ctrl_bf1_process1"
  ctrl_gen/1(data_out) -> hta_est_data/1  "OFDM_bf1_process1"
  Product/1 -> ctrl_gen/1(data_in)
  cos + jsin/1 -> Switch/1
  Data Type Conversion3/1 -> cos + jsin/1

== system rx2/demode1/chan_est1/Subsystem/HDL_DUT2/delta_estimator ==
  data_in : Inport
  valid_in : Inport  Port=2  OutDataTypeStr=boolean
  Add1 : Sum  Inputs=+-  AccumDataTypeStr=fixdt(1,64,56)  OutDataTypeStr=fixdt(1,32,28)
  Delay2 : Delay  DelayLength=1  InitialCondition=0
  calculate_norm2 : Subsystem
  calculate_norm3 : Subsystem
  iteration_estimation : Subsystem
  iteration_estimation1 : Subsystem
  data_out : Outport  OutDataTypeStr=fixdt(1,16,14)  VectorParamsAs1DForOutWhenUnconnected=off
  valid_out : Outport  Port=2  OutDataTypeStr=boolean  VectorParamsAs1DForOutWhenUnconnected=off
  wires:
  valid_in/1 -> iteration_estimation/2(valid_in)
  iteration_estimation/1(data_out) -> calculate_norm3/1(data_in)
  calculate_norm2/1(data_out) -> Add1/1
  calculate_norm3/1(data_out) -> Add1/2
  Add1/1 -> iteration_estimation1/1(data_in)
  data_in/1 -> Delay2/1, iteration_estimation/1(data_in)
  iteration_estimation1/1(data_out) -> data_out/1
  iteration_estimation1/2(valid_out) -> valid_out/1
  Delay2/1 -> calculate_norm2/1(data_in)
  iteration_estimation/2(valid_out) -> iteration_estimation1/2(valid_in)

== system rx2/demode1/chan_est1/Subsystem/HDL_DUT3/H_est ==
  H_result_in : Inport
      settings: SignalType=complex
  H_ctrl_in : Inport  Port=2  OutDataTypeStr=Bus: samplecontrol
  Complex to Real-Imag : ComplexToRealImag
  Constant1 : Constant  OutDataTypeStr=fixdt(1,33,28)
  Constant2 : Constant  Value=2  OutDataTypeStr=uint8
  Counter1 : hdlsllib/Sources/HDL Counter  CountType=Count limited  CountInit=0  CountStep=1  CountMax=1  CountFromType=Initial value  CountFrom=0  CountResetPort=off  CountLoadPort=off  CountEnbPort=on  CountDirPort=off  CountHitOutputPort=off  CountDataType=Unsigned  CountWordLen=8  CountFracLen=0  CountSampTime=1
  Counter2 : hdlsllib/Sources/HDL Counter  CountType=Count limited  CountInit=0  CountStep=1  CountMax=511  CountFromType=Initial value  CountFrom=0  CountResetPort=off  CountLoadPort=off  CountEnbPort=on  CountDirPort=off  CountHitOutputPort=off  CountDataType=Unsigned  CountWordLen=16  CountFracLen=0  CountSampTime=1
  Counter3 : hdlsllib/Sources/HDL Counter  CountType=Count limited  CountInit=0  CountStep=1  CountMax=511  CountFromType=Initial value  CountFrom=0  CountResetPort=on  CountLoadPort=off  CountEnbPort=on  CountDirPort=off  CountHitOutputPort=off  CountDataType=Unsigned  CountWordLen=16  CountFracLen=0  CountSampTime=1
  Counter4 : hdlsllib/Sources/HDL Counter  CountType=Count limited  CountInit=0  CountStep=1  CountMax=5  CountFromType=Initial value  CountFrom=0  CountResetPort=on  CountLoadPort=off  CountEnbPort=on  CountDirPort=off  CountHitOutputPort=on  CountDataType=Unsigned  CountWordLen=16  CountFracLen=0  CountSampTime=1
  Delay1 : Delay  DelayLength=1  InitialCondition=0
  Delay2 : Delay  DelayLength=12  InitialCondition=0
  Delay3 : Delay  DelayLength=1  InitialCondition=0
  Delay4 : Delay  DelayLength=1  InitialCondition=0
  Delay5 : Delay  DelayLength=12  InitialCondition=0
  Delay6 : Delay  DelayLength=12  InitialCondition=0
  Gain3 : Gain  Gain=1/6  OutDataTypeStr=fixdt(1,32,27)
  Ground{1..6} (6 alike) : Ground
  Logical Operator : Logic  Operator=XOR  AllPortsSameDT=off  OutDataTypeStr=boolean
  Logical Operator2 : Logic  Operator=OR  AllPortsSameDT=off  OutDataTypeStr=boolean
  Mod : Math  Operator=mod  SignedPower=on
  MultiplyAccumulate : hdlsllib/HDL Operations/Multiply-Accumulate  opMode=Streaming - using Number of Samples  initValueSetting=Dialog  initValue=0  initValueSetting2=Dialog  initValue2=0  initValueSetting3=Dialog  initValue3=0  num_samples=6  RndMeth2=Floor  RndMeth3=Floor  datatype2=Inherit: Inherit via back propagation  datatype3=Inherit: Inherit via back propagation  validOut=on  endInandOut=on  startOut=on  countOut=on  dim=-1  DoSatur=off  parallel=off
  MultiplyAccumulate1 : hdlsllib/HDL Operations/Multiply-Accumulate  opMode=Streaming - using Number of Samples  initValueSetting=Dialog  initValue=0  initValueSetting2=Dialog  initValue2=0  initValueSetting3=Dialog  initValue3=0  num_samples=6  RndMeth2=Floor  RndMeth3=Floor  datatype2=Inherit: Inherit via back propagation  datatype3=Inherit: Inherit via back propagation  validOut=on  endInandOut=on  startOut=on  countOut=on  dim=-1  DoSatur=off  parallel=off
  Real-Imag to Complex : RealImagToComplex
  Sample Control Bus Creator : whdlutilities/Sample Control Bus Creator
  Sample Control Bus Selector : whdlutilities/Sample Control Bus Selector  OutputSignals=start,end,valid
  Switch1 : Switch  Threshold=396  SaturateOnIntegerOverflow=off  InputSameDT=off
  Switch2 : Switch  Threshold=1  SaturateOnIntegerOverflow=off  InputSameDT=off
  Switch3 : Switch  Threshold=5  SaturateOnIntegerOverflow=off  InputSameDT=off
  Switch4 : Switch  Threshold=396  SaturateOnIntegerOverflow=off  InputSameDT=off
  Switch5 : Switch  Threshold=396  SaturateOnIntegerOverflow=off  InputSameDT=off
  Switch6 : Switch  Threshold=5  SaturateOnIntegerOverflow=off  InputSameDT=off
  hRAM1 : Subsystem
  H_out : Outport  VectorParamsAs1DForOutWhenUnconnected=off
  H_valid_out : Outport  Port=2  VectorParamsAs1DForOutWhenUnconnected=off
  wires:
  Switch4/1 -> Switch3/1  "H_sum"
  Sample Control Bus Selector/2 -> Logical Operator2/1, Delay4/1
  Sample Control Bus Selector/1 -> Delay3/1, Logical Operator2/2, Counter3/1
  Logical Operator/1 -> Switch2/2, Switch1/3, Counter3/2, Counter2/1  "valid_1024"
  Switch2/1 -> MultiplyAccumulate/1
  Counter1/1 -> Mod/1
  Ground1/1 -> Switch2/3
  Counter3/1 -> Switch5/2, Switch4/2
  Ground4/1 -> Switch1/1
  Ground2/1 -> Switch3/3
  MultiplyAccumulate/1 -> Switch4/3
  H_ctrl_in/1 -> Sample Control Bus Selector/1
  Delay1/1 -> Delay5/1, hRAM1/2(H_valid_out)
  Ground3/1 -> Switch4/1
  Logical Operator2/1 -> Counter4/1
  Switch1/1 -> MultiplyAccumulate1/3, Counter4/2  "valid_792"
  Constant2/1 -> Mod/2
  Counter4/1 -> Switch6/2, Switch3/2
  Counter2/1 -> Switch1/2
  Delay3/1 -> Delay2/1
  Mod/1 -> Logical Operator/2
  Constant1/1 -> MultiplyAccumulate1/2, MultiplyAccumulate/2
  Delay4/1 -> hRAM1/3(H_end_out), Delay6/1
  hRAM1/1(Out1) -> H_out/1
  Sample Control Bus Selector/3 -> Counter1/1, Logical Operator/1, Delay1/1
  Sample Control Bus Creator/1 -> H_valid_out/1
  H_result_in/1 -> Complex to Real-Imag/1
  MultiplyAccumulate1/1 -> Switch5/3
  Ground5/1 -> Switch5/1
  Switch5/1 -> Switch6/1  "H_sum"
  Ground6/1 -> Switch6/3
  Complex to Real-Imag/1 -> MultiplyAccumulate1/1
  Complex to Real-Imag/2 -> Switch2/1
  Gain3/1 -> hRAM1/1(H_out)  "average"
  Switch6/1 -> Real-Imag to Complex/1
  Switch3/1 -> Real-Imag to Complex/2
  Real-Imag to Complex/1 -> Gain3/1
  Delay2/1 -> Sample Control Bus Creator/1
  Delay5/1 -> Sample Control Bus Creator/3
  Delay6/1 -> Sample Control Bus Creator/2

== system rx2/demode1/chan_est1/Subsystem/HDL_DUT3/LS_Est ==
  LS_data_in : Inport
  LS_polit_in : Inport  Port=2  OutDataTypeStr=fixdt(1,16,14)
  LS_valid_in : Inport  Port=3
  Complex to Magnitude-Angle : dsphdlmathfun2/Complex to Magnitude-Angle  NumIterationsSource=Property  NumIterations=10  OutputFormat=Magnitude and angle  AngleFormat=Normalized  ScaleOutput=on  ScalingMethod=Multiplier  SimulateUsing=Code generation
  Complex to Magnitude-Angle1 : dsphdlmathfun2/Complex to Magnitude-Angle  NumIterationsSource=Property  NumIterations=10  OutputFormat=Magnitude and angle  AngleFormat=Normalized  ScaleOutput=on  ScalingMethod=Shift-Add  SimulateUsing=Code generation
  Dot Product : DotProduct  OutDataTypeStr=fixdt(1,16,12)
  Ground : Ground
  Ground1 : Ground
  HDL Counter : hdlsllib/Sources/HDL Counter  CountType=Count limited  CountInit=0  CountStep=1  CountMax=1  CountFromType=Initial value  CountFrom=0  CountResetPort=off  CountLoadPort=off  CountEnbPort=on  CountDirPort=off  CountHitOutputPort=off  CountDataType=Unsigned  CountWordLen=2  CountFracLen=0  CountSampTime=1
  Switch1 : Switch  Threshold=1  OutDataTypeStr=fixdt(1,16,14)  SaturateOnIntegerOverflow=off  InputSameDT=off
  Switch2 : Switch  Threshold=1  OutDataTypeStr=fixdt(1,16,14)  SaturateOnIntegerOverflow=off  InputSameDT=off
  ctrl_gen : Subsystem
  ctrl_gen1 : Subsystem
  LS_result_out : Outport  VectorParamsAs1DForOutWhenUnconnected=off
  LS_ctrl_out : Outport  Port=2  VectorParamsAs1DForOutWhenUnconnected=off
  wdata_out : Outport  Port=3  VectorParamsAs1DForOutWhenUnconnected=off
  wvalid_out : Outport  Port=4  VectorParamsAs1DForOutWhenUnconnected=off
  wires:
  LS_data_in/1 -> Switch1/1, Switch2/1
  Switch1/1 -> Dot Product/1  "data"
  Dot Product/1 -> Complex to Magnitude-Angle/1
  Ground/1 -> Switch1/3
  LS_valid_in/1 -> Complex to Magnitude-Angle/2, Complex to Magnitude-Angle1/2, HDL Counter/1, Switch1/2
  LS_polit_in/1 -> Dot Product/2
  Complex to Magnitude-Angle/1 -> ctrl_gen/1(data_in)  "result"
  Complex to Magnitude-Angle/3 -> ctrl_gen/2(valid_in)  "valid2"
  ctrl_gen/1(data_out) -> LS_result_out/1
  ctrl_gen/2(ctrl_out) -> LS_ctrl_out/1
  HDL Counter/1 -> Switch2/2
  Ground1/1 -> Switch2/3
  Switch2/1 -> Complex to Magnitude-Angle1/1  "data"
  Complex to Magnitude-Angle1/1 -> wdata_out/1
  Complex to Magnitude-Angle1/3 -> ctrl_gen1/1(valid_in)
  ctrl_gen1/1(wvalid_out) -> wvalid_out/1

== system rx2/demode1/chan_est1/Subsystem/HDL_DUT3/Pliot ==
  enb : Inport
  Counter1 : hdlsllib/Sources/HDL Counter  CountType=Count limited  CountInit=0  CountStep=1  CountMax=7  CountFromType=Initial value  CountFrom=0  CountResetPort=off  CountLoadPort=off  CountEnbPort=on  CountDirPort=off  CountHitOutputPort=off  CountDataType=Unsigned  CountWordLen=8  CountFracLen=0  CountSampTime=1
  Data Type Conversion3 : DataTypeConversion  OutDataTypeStr=uint8  SaturateOnIntegerOverflow=off  RndMeth=Floor
  rom : Subsystem
  pilot : Outport
  wires:
  enb/1 -> Counter1/1
  Counter1/1 -> Data Type Conversion3/1
  Data Type Conversion3/1 -> rom/1(address)
  rom/1(data_out) -> pilot/1  "pilot"

== system rx2/demode1/chan_est1/Subsystem/HDL_DUT3/TA_EST ==
  data_in : Inport
  ctrl_in : Inport  Port=2  OutDataTypeStr=Bus: samplecontrol
  Bus Selector : BusSelector  OutputSignals=start,end,valid
  Complex to Magnitude-Angle : dsphdlmathfun2/Complex to Magnitude-Angle  NumIterationsSource=Property  NumIterations=10  OutputFormat=Magnitude and angle  AngleFormat=Radians  ScaleOutput=on  ScalingMethod=Shift-Add  SimulateUsing=Code generation
  Constant : Constant  OutDataTypeStr=fixdt(1,34,24)
  Counter1 : hdlsllib/Sources/HDL Counter  CountType=Count limited  CountInit=0  CountStep=1  CountMax=1  CountFromType=Initial value  CountFrom=0  CountResetPort=off  CountLoadPort=off  CountEnbPort=on  CountDirPort=off  CountHitOutputPort=off  CountDataType=Unsigned  CountWordLen=8  CountFracLen=0  CountSampTime=1
  Counter2 : hdlsllib/Sources/HDL Counter  CountType=Count limited  CountInit=0  CountStep=1  CountMax=511  CountFromType=Initial value  CountFrom=0  CountResetPort=off  CountLoadPort=off  CountEnbPort=on  CountDirPort=off  CountHitOutputPort=off  CountDataType=Unsigned  CountWordLen=16  CountFracLen=0  CountSampTime=1
  Counter3 : hdlsllib/Sources/HDL Counter  CountType=Count limited  CountInit=0  CountStep=1  CountMax=5  CountFromType=Initial value  CountFrom=0  CountResetPort=off  CountLoadPort=off  CountEnbPort=on  CountDirPort=off  CountHitOutputPort=on  CountDataType=Unsigned  CountWordLen=8  CountFracLen=0  CountSampTime=1
  Counter4 : hdlsllib/Sources/HDL Counter  CountType=Count limited  CountInit=0  CountStep=1  CountMax=395  CountFromType=Initial value  CountFrom=0  CountResetPort=off  CountLoadPort=off  CountEnbPort=on  CountDirPort=off  CountHitOutputPort=off  CountDataType=Unsigned  CountWordLen=16  CountFracLen=0  CountSampTime=1
  Data Type Conversion : DataTypeConversion  OutDataTypeStr=boolean  SaturateOnIntegerOverflow=off  RndMeth=Floor
  Data Type Conversion1 : DataTypeConversion  OutDataTypeStr=fixdt(1,26,14)  SaturateOnIntegerOverflow=off  RndMeth=Floor
  Data Type Conversion2 : DataTypeConversion  OutDataTypeStr=fixdt(1,26,14)  SaturateOnIntegerOverflow=off  RndMeth=Floor
  Data Type Conversion3 : DataTypeConversion  OutDataTypeStr=fixdt(1,16,14)  SaturateOnIntegerOverflow=off  RndMeth=Floor
  Delay1 : Delay  InitialCondition=0
  Delay2 : Delay  InitialCondition=0
  Delay3 : Delay  DelayLength=1  InitialCondition=0
  Delay4 : Delay  DelayLength=3  InitialCondition=0
  Delay5 : Delay  DelayLength=18  InitialCondition=0
  Delay6 : Delay  DelayLength=15  InitialCondition=0
  Delay7 : Delay  DelayLength=1  InitialCondition=0
  Dot Product : DotProduct  OutDataTypeStr=Inherit: Inherit via internal rule
  Dot Product1 : DotProduct  OutDataTypeStr=fixdt(1,26,14)
  Ground : Ground
  Ground4 : Ground
  Logical Operator : Logic  Operator=XOR  AllPortsSameDT=off  OutDataTypeStr=boolean
  Logical Operator1 : Logic  AllPortsSameDT=off  OutDataTypeStr=boolean
  Logical Operator2 : Logic  Operator=XOR  AllPortsSameDT=off  OutDataTypeStr=boolean
  Multiply-Accumulate : hdlsllib/HDL Operations/Multiply-Accumulate  opMode=Streaming - using Number of Samples  initValueSetting=Dialog  initValue=0  initValueSetting2=Dialog  initValue2=0  initValueSetting3=Dialog  initValue3=0  num_samples=330  RndMeth2=Floor  RndMeth3=Floor  datatype2=Inherit: Inherit via back propagation  datatype3=fixdt(1,68,48)  validOut=on  endInandOut=on  startOut=on  countOut=on  dim=-1  DoSatur=off  parallel=off
  Product : Product
  Switch : Switch  Criteria=u2 ~= 0  OutDataTypeStr=fixdt(1,26,14)  SaturateOnIntegerOverflow=off  InputSameDT=off
  Switch1 : Switch  Threshold=396  SaturateOnIntegerOverflow=off  InputSameDT=off
  cos + jsin : Trigonometry  Operator=cos + jsin  ApproximationMethod=CORDIC  NumberOfIterations=10
  ctrl_gen : Subsystem
  hta_est_data : Outport  VectorParamsAs1DForOutWhenUnconnected=off
  hta_est_ctrl : Outport  Port=2  VectorParamsAs1DForOutWhenUnconnected=off
  wires:
  ctrl_in/1 -> Bus Selector/1
  data_in/1 -> Delay5/1, Dot Product/1, Delay1/1
  Dot Product/1 -> Multiply-Accumulate/1
  Delay1/1 -> Dot Product/2
  Constant/1 -> Multiply-Accumulate/2
  Multiply-Accumulate/1 -> Complex to Magnitude-Angle/1
  Ground4/1 -> Switch1/1
  Counter2/1 -> Switch1/2
  Logical Operator/1 -> Switch1/3, Counter2/1  "valid_1024"
  Counter1/1 -> Data Type Conversion/1
  Delay2/1 -> Logical Operator/1, Counter1/1
  Switch1/1 -> Delay6/1, Logical Operator2/1, Counter3/1  "valid_792"
  Data Type Conversion/1 -> Logical Operator/2
  Counter3/2 -> Logical Operator1/2, Delay3/1
  Delay3/1 -> Logical Operator1/1
  Logical Operator1/1 -> Logical Operator2/2
  Logical Operator2/1 -> Multiply-Accumulate/3
  Delay4/1 -> Complex to Magnitude-Angle/2
  Complex to Magnitude-Angle/3 -> Delay7/1
  Delay6/1 -> Counter4/1
  Complex to Magnitude-Angle/2 -> Data Type Conversion2/1
  Counter4/1 -> Data Type Conversion1/1
  Data Type Conversion1/1 -> Dot Product1/2
  Dot Product1/1 -> Data Type Conversion3/1
  Data Type Conversion2/1 -> Dot Product1/1
  Switch/1 -> Product/2
  Ground/1 -> Switch/3
  Delay7/1 -> ctrl_gen/2(valid_in), Switch/2
  Delay5/1 -> Product/1
  Bus Selector/3 -> [valid], Delay4/1, Delay2/1  "<valid>"
  ctrl_gen/2(ctrl_out) -> hta_est_ctrl/1  "OFDM_ctrl_bf1_process1"
  ctrl_gen/1(data_out) -> hta_est_data/1  "OFDM_bf1_process1"
  Product/1 -> ctrl_gen/1(data_in)
  cos + jsin/1 -> Switch/1
  Data Type Conversion3/1 -> cos + jsin/1

== system rx2/demode1/chan_est1/Subsystem/HDL_DUT3/delta_estimator ==
  data_in : Inport
  valid_in : Inport  Port=2  OutDataTypeStr=boolean
  Add1 : Sum  Inputs=+-  AccumDataTypeStr=fixdt(1,64,56)  OutDataTypeStr=fixdt(1,32,28)
  Delay2 : Delay  DelayLength=1  InitialCondition=0
  calculate_norm2 : Subsystem
  calculate_norm3 : Subsystem
  iteration_estimation : Subsystem
  iteration_estimation1 : Subsystem
  data_out : Outport  OutDataTypeStr=fixdt(1,16,14)  VectorParamsAs1DForOutWhenUnconnected=off
  valid_out : Outport  Port=2  OutDataTypeStr=boolean  VectorParamsAs1DForOutWhenUnconnected=off
  wires:
  valid_in/1 -> iteration_estimation/2(valid_in)
  iteration_estimation/1(data_out) -> calculate_norm3/1(data_in)
  calculate_norm2/1(data_out) -> Add1/1
  calculate_norm3/1(data_out) -> Add1/2
  Add1/1 -> iteration_estimation1/1(data_in)
  data_in/1 -> Delay2/1, iteration_estimation/1(data_in)
  iteration_estimation1/1(data_out) -> data_out/1
  iteration_estimation1/2(valid_out) -> valid_out/1
  Delay2/1 -> calculate_norm2/1(data_in)
  iteration_estimation/2(valid_out) -> iteration_estimation1/2(valid_in)
